simulink model "CDC2025_HybridAutomaton"  (R2023b)
settings: Solver=VariableStepAuto  StartTime=0.0  StopTime=sim_T  MaxStep=MaxStep  RelTol=RelTol
values from neighbouring files (symbols this model uses):
  A_sim = double(jacobian(dx, x))    [Settings_Simulation.m]
  B_sim = double(jacobian(dx, ui))    [Settings_Simulation.m]
  sim_T = 10    [MAIN_Simulation.m]
undefined symbols (not defined in the file or in its folder): control, leader, model, simulation
libraries: HyEQ_Library x1
settings Model: Creator=20155555  LastModifiedBy=20155555
settings OptimizationCC: BlockReduction=off  DefaultParameterBehavior=Inlined  BufferReuse=off

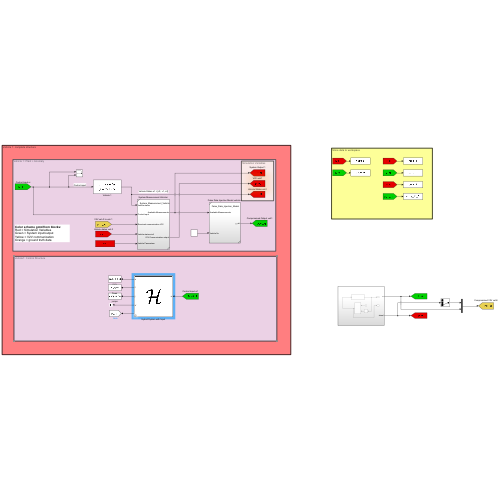
[thumbnail: Simulink's stored preview of the top-level diagram]
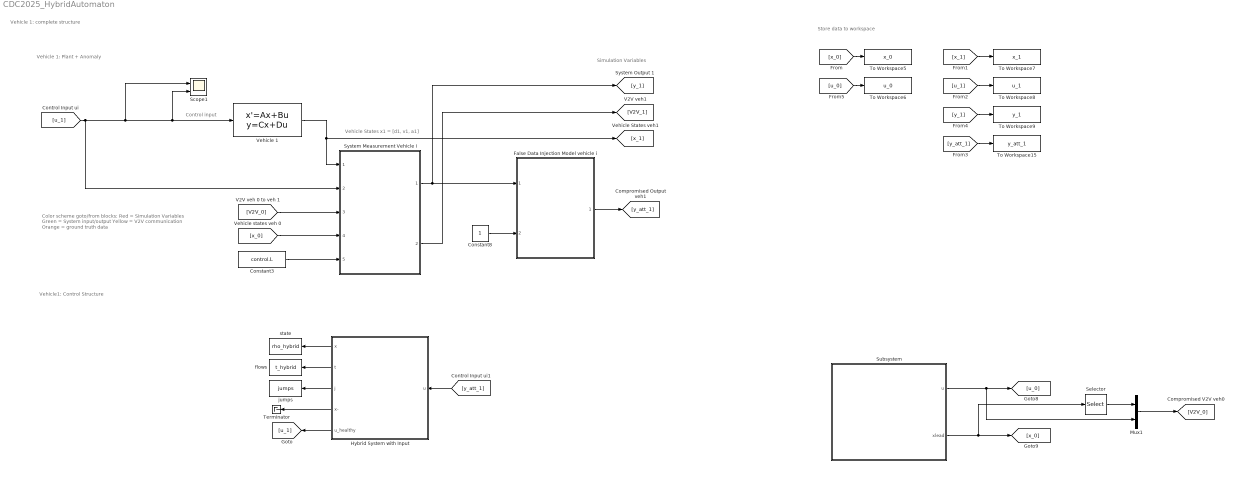
== system CDC2025_HybridAutomaton ==
  note: Vehicle 1: complete structure
  note: Vehicle1: Control Structure
  note: Vehicle States x1 = [d1, v1, a1]
  note: Store data to workspace
  note: Control input
  note: Vehicle 1: Plant + Anomaly
  note: Simulation Variables
  note: Color scheme goto/from blocks:
      | Red = Simulation Variables
      | Green = System input/output
      | Yellow = V2V communication
      | Orange = ground truth data
  Constant3 : Constant  Value=control.L
  Constant8 : Constant
  False Data Injection Model vehicle i : Subsystem  ReferencedSubsystem=False_Data_Injection_Model
  Hybrid System with Input : Subsystem  LoadFcn=set_param(gcb,'LinkStatus','none')  mask(Hybrid System with Inputs){x0=simulation.rho_init, input_dim=6, parameters=[control.h, model.tau, control.kp, control.kd, control.epsilon], T=sim_T, J=control.J, rule=Flow}
      mask prompts: x0 "Initial Condition (column vector)"; input_dim "Input Dimension (positive integer)"; T "Flow Horizon (nonnegative real)"; J "Jump Horizon (nonnegative integer)"; rule "Flow/Jump Priorty Rule"
      mask help:
      | To modify (f, g, C, D) for this block, "Look inside" the block mask by either clicking the down arrow in the lower-left corner or selecting "Mask" > "Look Under Mask" from the context menu.
      |
      | For instructions how to use this block, see the
      mask init:
      | state_dim = numel(x0);
      settings: CopyFcn=|
      | set_param(gcb,'LinkStatus','none'),
      | set_param(gcs, 'MaxStep', 'MaxStep', 'RelTol', 'RelTol','StopTime', 'T')
      mask Help:
      | To modify (f, g, C, D) for this block, "Look inside" the block mask by either clicking the down arrow in the lower-left corner or selecting "Mask" > "Look Under Mask" from the context menu.
      | 
      | The value given in the 'parameters' field is passed as the last input argument for f, g, C, and D. Any MATLAB object can be used, but we recommend using a struct. For example, in the initialization script, a parameters struct can be defined as followed.
      |   parameters = struct();
      |   parameters.A = eye(2);
      |   parameters.B = [1; 0];
      | 
      | The output "x-" is the state output delayed by one integration step. Use this output to break algebraic loops.
      mask TypeOptions x0: Integrator System/x0
      mask TypeOptions T: Integrator System/T
      mask TypeOptions J: Integrator System/J
      mask TypeOptions rule: Jump | Flow | Random
      mask DialogControl Control2 Prompt: Introduction to the HyEQ Simulink-based Library
      mask DialogControl Control2 Callback: hybrid.internal.openHelp('Help_SimulinkLibrary')
      mask DialogControl Container3 Prompt: System Configuration
      mask DialogControl Container2 Prompt: Solver Options
      mask Display:
      | image('Hcal.jpg')
      | port_label('output', 1, 'x')
      | port_label('output', 2, 't')
      | port_label('output', 3, 'j')
      | port_label('output', 4, 'x^-','texmode', 'on')
      | port_label('input', 1, 'u')
  Mux1 : Mux  Inputs=2
  Scope1 : Scope  NumInputPorts=2
  Selector : Selector  InputPortWidth=3  IndexOptions=Index vector (dialog)  Indices=[3]  OutputSizes=1
  Subsystem : Subsystem
  System Measurement Vehicle i : Subsystem  ReferencedSubsystem=System_Measurement_Vehicle
  Terminator : Terminator
  To Workspace15 : ToWorkspace  VariableName=y_att_1  SampleTime=-1
  To Workspace5 : ToWorkspace  VariableName=x_0  SampleTime=-1
  To Workspace6 : ToWorkspace  VariableName=u_0  SampleTime=-1
  To Workspace7 : ToWorkspace  VariableName=x_1  SampleTime=-1
  To Workspace8 : ToWorkspace  VariableName=u_1  SampleTime=-1
  To Workspace9 : ToWorkspace  VariableName=y_1  SampleTime=-1
  Vehicle 1 : StateSpace  A=A_sim  B=B_sim  C=eye(3)  D=zeros(3,1)  InitialCondition=simulation.veh1.x_init
  flows : ToWorkspace  VariableName=t_hybrid  SampleTime=-1
  jumps : ToWorkspace  VariableName=jumps  SampleTime=-1
  state : ToWorkspace  VariableName=rho_hybrid  SampleTime=-1
  wires:
  Hybrid System with Input/4(x-) -> Terminator/1
  Hybrid System with Input/1(x) -> state/1
  Hybrid System with Input/2(t) -> flows/1
  Hybrid System with Input/3(j) -> jumps/1
  Hybrid System with Input/5(u_healthy) -> [u_1]
  Constant8/1 -> False Data Injection Model vehicle i/2
  False Data Injection Model vehicle i/1 -> [y_att_1]
  [V2V_0] -> System Measurement Vehicle i/3
  [x_0] -> To Workspace5/1
  [y_att_1] -> To Workspace15/1
  Mux1/1 -> [V2V_0]
  [u_1] -> To Workspace8/1
  [x_1] -> To Workspace7/1
  [y_1] -> To Workspace9/1
  System Measurement Vehicle i/2 -> [V2V_1]
  [x_0] -> System Measurement Vehicle i/4
  [u_1] -> Vehicle 1/1, Scope1/2, Scope1/1, System Measurement Vehicle i/2
  Subsystem/2(xlead) -> Selector/1, [x_0]
  [u_0] -> To Workspace6/1
  Subsystem/1(u) -> Mux1/2, [u_0]
  Selector/1 -> Mux1/1
  Vehicle 1/1 -> System Measurement Vehicle i/1, [x_1]
  Constant3/1 -> System Measurement Vehicle i/5
  System Measurement Vehicle i/1 -> [y_1], False Data Injection Model vehicle i/1
  [y_att_1] -> Hybrid System with Input/1(u)

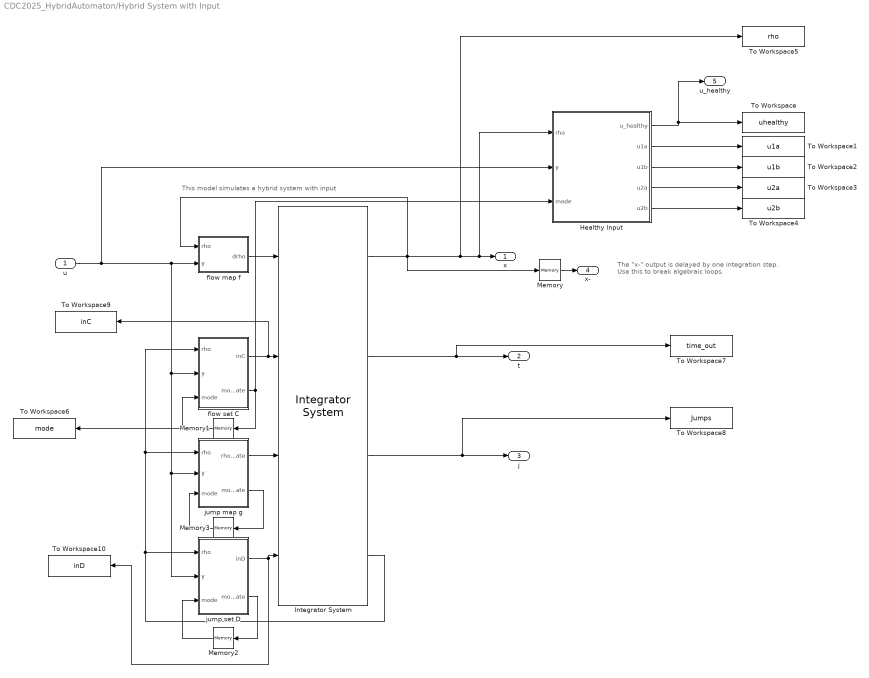
== system CDC2025_HybridAutomaton/Hybrid System with Input ==
  note: This model simulates a hybrid system with input
  note: The "x-" output is delayed by one integration step. Use this to break algebraic loops.
  u : Inport  PortDimensions=input_dim
  Healthy Input : MATLAB Function  TreatAsAtomicUnit=on
  Integrator System : HyEQ_Library/Other/Integrator System  Priority=2  T=T  J=J  x0=x0  rule=rule
      settings: SourceProductName=Hybrid Equations Toolbox
  Memory : Memory  InitialCondition=x0
  Memory1 : Memory  InheritSampleTime=on
  Memory2 : Memory  InheritSampleTime=on
  Memory3 : Memory  InheritSampleTime=on
  To Workspace : ToWorkspace  VariableName=uhealthy  SampleTime=-1
  To Workspace1 : ToWorkspace  VariableName=u1a  SampleTime=-1
  To Workspace10 : ToWorkspace  VariableName=inD  SampleTime=-1
  To Workspace2 : ToWorkspace  VariableName=u1b  SampleTime=-1
  To Workspace3 : ToWorkspace  VariableName=u2a  SampleTime=-1
  To Workspace4 : ToWorkspace  VariableName=u2b  SampleTime=-1
  To Workspace5 : ToWorkspace  VariableName=rho  SampleTime=-1
  To Workspace6 : ToWorkspace  VariableName=mode  SampleTime=-1
  To Workspace7 : ToWorkspace  VariableName=time_out  SampleTime=-1
  To Workspace8 : ToWorkspace  VariableName=Jumps  SampleTime=-1
  To Workspace9 : ToWorkspace  VariableName=inC  SampleTime=-1
  flow map f : MATLAB Function  TreatAsAtomicUnit=on
  flow set C : MATLAB Function  TreatAsAtomicUnit=on
  jump map g : MATLAB Function  TreatAsAtomicUnit=on
  jump set D : MATLAB Function  TreatAsAtomicUnit=on
  x : Outport  PortDimensions=state_dim
  t : Outport  Port=2  PortDimensions=1
  j : Outport  Port=3  PortDimensions=1
  x- : Outport  Port=4  PortDimensions=state_dim
  u_healthy : Outport  Port=5
  wires:
  Memory/1 -> x-/1
  jump map g/1(rho_update) -> Integrator System/3
  jump set D/1(inD) -> Integrator System/4, To Workspace10/1
  u/1 -> Healthy Input/2(y), jump set D/2(y), jump map g/2(y), flow set C/2(y), flow map f/2(y)
  Integrator System/3 -> To Workspace8/1, j/1
  Integrator System/2 -> To Workspace7/1, t/1
  flow set C/1(inC) -> To Workspace9/1, Integrator System/2
  Integrator System/1 -> flow map f/1(rho), To Workspace5/1, Healthy Input/1(rho), x/1, Memory/1
  Integrator System/4 -> flow set C/1(rho), jump map g/1(rho), jump set D/1(rho)
  flow map f/1(drho) -> Integrator System/1
  Memory1/1 -> flow set C/3(mode), To Workspace6/1
  Memory2/1 -> jump set D/3(mode)
  jump set D/2(mode_update) -> Memory2/1
  Memory3/1 -> jump map g/3(mode)
  jump map g/2(mode_update) -> Memory3/1
  Healthy Input/1(u_healthy) -> u_healthy/1, To Workspace/1
  Healthy Input/2(u1a) -> To Workspace1/1
  Healthy Input/5(u2b) -> To Workspace4/1
  Healthy Input/4(u2a) -> To Workspace3/1
  Healthy Input/3(u1b) -> To Workspace2/1
  flow set C/2(mode_update) -> Memory1/1, Healthy Input/3(mode)

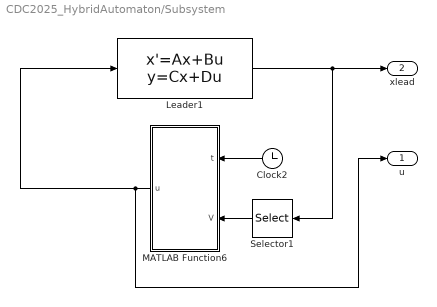
== system CDC2025_HybridAutomaton/Subsystem ==
  Clock2 : Clock
  Leader1 : StateSpace  A=A_sim  B=B_sim  C=eye(3)  D=zeros(3,1)  InitialCondition=simulation.veh0.x_init
  MATLAB Function6 : MATLAB Function  TreatAsAtomicUnit=on
  Selector1 : Selector  InputPortWidth=3  IndexOptions=Index vector (dialog)  Indices=2  OutputSizes=1
  u : Outport
  xlead : Outport  Port=2
  wires:
  Selector1/1 -> MATLAB Function6/2(V)
  MATLAB Function6/1(u) -> u/1, Leader1/1
  Leader1/1 -> xlead/1, Selector1/1
  Clock2/1 -> MATLAB Function6/1(t)

== matlab function CDC2025_HybridAutomaton/Subsystem/MATLAB Function6 ==
  data: t input; u output; V input; control parameter; leader parameter
function u = fcn(t, V, control, leader)


kp = control.kp;

Vdes = leader.Vdes0 ;
u = kp*(Vdes - V);

end

== matlab function CDC2025_HybridAutomaton/Hybrid System with Input/Healthy Input ==
  data: rho input size=state_dim; y input size=input_dim; mode input; u_healthy output size=1; parameters parameter; u1a output; u1b output; u2a output; u2b output
function [u_healthy, u1a, u1b, u2a, u2b]  = uHealthy(rho, y, mode, parameters)
% Define flow set indictor function here.

% allocate state
rho1a = rho(1);
rho1b = rho(2);
rho2a = rho(3);
rho2b = rho(4);

% Allocate output
y1 = y(1);
y2 = y(2);
y5a = y(3);
y5b = y(4);
y6a = y(5);
y6b = y(6);

% parameters
h = parameters(1);
tau = parameters(2);
kp = parameters(3);
kd = parameters(4);

% Compute control inputs before reset
u1a = compute_u1(y1, y2, y5a, rho1a, kd, h, tau);
u1b = compute_u1(y1, y2, y5b, rho1b, kd, h, tau);
u2a = compute_u2(y1, y2, rho2a, kd, h);
u2b = compute_u2(y1, y2, rho2b, kd, h);


if mode == 0
    u_healthy = u1a;
elseif mode ==  1
    u_healthy = u1b;
elseif mode == 2
    u_healthy = u1a;
elseif mode == 3
    u_healthy = u1a;
elseif mode == 4
    u_healthy = u1a;
else
    u_healthy = 69;
end

end



function u = compute_u1(y1, y2, y5, rho, kd, h, tau)
% Compute control input u1
u = rho + (kd/h) * y1 - kd * y2 + (tau/h) * y5;
end

function u = compute_u2(y1, y2, rho, kd, h)
% Compute control input u2
u = rho + (kd/h) * y1 - kd * y2;
end

== matlab function CDC2025_HybridAutomaton/Hybrid System with Input/flow map f ==
  data: rho input size=state_dim; y input size=input_dim; drho output size=state_dim; parameters parameter
function drho = f(rho, y, parameters)
% Define flow map here.

% parameters
h = parameters(1);
tau = parameters(2);
kp = parameters(3);
kd = parameters(4);

% States
rho1a = rho(1);
rho1b = rho(2);
rho2a = rho(3);
rho2b = rho(4);

% input
y1 = y(1);
y2 = y(2);
y5a = y(3);
y5b = y(4);
y6a = y(5);
y6b = y(6);

% Update states (flow dynamics)
drho1a = update_drho1(rho1a, y1, y2, y5a, h, kp, kd, tau);
drho1b = update_drho1(rho1b, y1, y2, y5b, h, kp, kd, tau);
drho2a = update_drho2(rho2a, y1, y2, y6a, h, kp, kd);
drho2b = update_drho2(rho2b, y1, y2, y6b, h, kp, kd);

drho = [drho1a; drho1b; drho2a; drho2b];

end


function drho = update_drho1(rho, y1, y2, y5, h, kp, kd, tau)
% Compute next state value
drho = (-1/h) * rho + (kp/h - kd/h^2) * y1 - (kp - kd/h) * y2 - (tau/h^2 - 1/h) * y5 - kp/h*3;
end

function drho = update_drho2(rho, y1, y2, y6, h, kp, kd)
% Compute next state value
drho = (-1/h) * rho + (kp/h - kd/h^2) * y1 - (kp - kd/h) * y2 + 1/h * y6 - kp/h*3;
end

== matlab function CDC2025_HybridAutomaton/Hybrid System with Input/flow set C ==
  data: rho input size=state_dim; y input size=input_dim; mode input; inC output size=1; parameters parameter; mode_update output
function [inC, mode_update] = C(rho, y, mode, parameters)
% Define flow set indictor function here.

% allocate state
rho1a = rho(1);
rho1b = rho(2);
rho2a = rho(3);
rho2b = rho(4);

% Allocate output
y1 = y(1);
y2 = y(2);
y5a = y(3);
y5b = y(4);
y6a = y(5);
y6b = y(6);

% parameters
h = parameters(1);
tau = parameters(2);
kp = parameters(3);
kd = parameters(4);
epsilon = parameters(5);

% Compute control inputs
u1a = compute_u1(y1, y2, y5a, rho1a, kd, h, tau);
u1b = compute_u1(y1, y2, y5b, rho1b, kd, h, tau);
u2a = compute_u2(y1, y2, rho2a, kd, h);
u2b = compute_u2(y1, y2, rho2b, kd, h);

% Determine transitions
[mode_update, inC, ~]  = get_next_mode(mode, u1a, u1b, u2a, u2b, y5a, y5b, y6a, y6b, rho1a, rho1b, rho2a, rho2b, h, tau, epsilon);



function [mode_update, inC, rho_update] = get_next_mode(mode, u1a, u1b, u2a, u2b, y5a, y5b, y6a, y6b, rho1a, rho1b, rho2a, rho2b, h, tau, epsilon)

% Compute next mode based on control inputs and state transitions
switch mode
    case 0
        if abs(u1a - u1b) > epsilon && abs(u1b - u2a) <= epsilon && abs(u2a - u2b) <= epsilon
            mode_update = 1;
            rho_update = [rho1a; rho1b; rho2a; rho2b];
            inC = false;
        elseif abs(u1b - u1a) > epsilon && abs(u1a - u2a) <= epsilon && abs(u2a - u2b) <= epsilon
            mode_update = 2;
            rho_update = [rho1a; rho1b; rho2a; rho2b];
            inC = false;
        elseif abs(u1a - u1b) <= epsilon && abs(u1b - u2b) <= epsilon && abs(u2b - u2a) > epsilon
            mode_update = 3;
            rho_update = [rho1a; rho1b; rho2a; rho2b];
            inC = false;
        elseif abs(u1a - u1b) <= epsilon && abs(u1b - u2a) <= epsilon && abs(u2a - u2b) > epsilon
            mode_update = 4;
            rho_update = [rho1a; rho1b; rho2a; rho2b];
            inC = false;
        else
            mode_update = mode;
            rho_update = [rho1a; rho1b; rho2a; rho2b];
            inC = true;
        end
    case 1 % Don't use u1a
        if abs(y5a - y5b) <= epsilon && abs(u1b - u2a) <= epsilon && abs(u2a - u2b) <= epsilon
            mode_update = 0;
            rho_update = [rho1b; rho1b; rho2a; rho2b];
            inC = false;
        elseif abs(u1b - u2a) > epsilon && abs(u2a - u2b) <= epsilon
            mode_update = 2;
            rho_update = [rho2a-tau/h*y5a; rho1b; rho2a; rho2b];
            inC = false;
        elseif abs(u1b - u2b) <= epsilon && abs(u2b - u2a) > epsilon
            mode_update = 3;
            rho_update = [rho1b; rho1b; rho2a; rho2b];
            % reset = 1;
            inC = false;
        elseif abs(u1b - u2a) <= epsilon && abs(u2a - u2b) > epsilon
            mode_update = 4;
            rho_update = [rho1b; rho1b; rho2a; rho2b];
            % reset = 1;
            inC = false;
        else
            mode_update = mode;
            rho_update = [rho1a; rho1b; rho2a; rho2b];
            inC = true;
        end
    case 2 % Don't use u1b
        if abs(y5a - y5b) <= epsilon && abs(u1a - u2a) <= epsilon && abs(u2a - u2b) <= epsilon
            mode_update = 0;
            rho_update = [rho1a; rho1a; rho2a; rho2b];
            inC = false;
        elseif abs(u1a - u2a) > epsilon && abs(u2a - u2b) <= epsilon
            mode_update = 1;
            rho_update = [rho1a; rho2a - tau/h*y5b; rho2a; rho2b];
            inC = false;
        elseif abs(u1a - u2a) > epsilon && abs(u1a - u2b) <= epsilon
            mode_update = 3;
            rho_update = [rho1a; rho1a; rho2a; rho2b];
            inC = false;
        elseif abs(u1a - u2a) <= epsilon && abs(u2a - u2b) > epsilon
            mode_update = 4;
            rho_update = [rho1a; rho1a; rho2a; rho2b];
            inC = false;
        else
            mode_update = mode;
            rho_update = [rho1a; rho1b; rho2a; rho2b];
            inC = true;
        end
    case 3 % Don't use u2a
        if abs(u1a - u1b) <= epsilon && abs(u1b - u2b) <= epsilon && abs(y6a - y6b) <= epsilon
            mode_update = 0;
            rho_update = [rho1a; rho1b; rho2b; rho2b];
            inC = false;
        elseif abs(u1a - u1b) > epsilon && abs(u1b - u2b) <= epsilon
            mode_update = 1;
            rho_update = [rho1a; rho1b; rho2b; rho2b];
            inC = false;
        elseif abs(u1b - u1a) > epsilon && abs(u1a - u2b) <= epsilon
            mode_update = 2;
            rho_update = [rho1a; rho1b; rho2b; rho2b];
            inC = false;
        elseif abs(u1a - u1b) <= epsilon && abs(u1b - u2b) > epsilon
            mode_update = 4;
            rho_update = [rho1a; rho1b; rho1a + tau/h*y5a; rho2b];
            inC = false;
        else
            mode_update = mode;
            rho_update = [rho1a; rho1b; rho2a; rho2b];
            inC = true;
        end
    case 4 % Don't use u2b
        if abs(u1a - u1b) <= epsilon && abs(u1b - u2a) <= epsilon && abs(y6a - y6b) <= epsilon
            mode_update = 0;
            rho_update = [rho1a; rho1b; rho2a; rho2a];
            inC = false;
        elseif abs(u1a - u1b) > epsilon && abs(u1b - u2a) <= epsilon
            mode_update = 1;
            rho_update = [rho1a; rho1b; rho2a; rho2a];
            inC = false;
        elseif abs(u1a - u1b) > epsilon && abs(u1a - u2a) <= epsilon
            mode_update = 2;
            rho_update = [rho1a; rho1b; rho2a; rho2a];
            inC = false;
        elseif abs(u1a - u1b) <= epsilon && abs(u1b - u2a) > epsilon
            mode_update = 3;
            rho_update = [rho1a; rho1b; rho2a; rho1a + tau/h*y5a];
            inC = false;
        else
            mode_update = mode;
            rho_update = [rho1a; rho1b; rho2a; rho2b];
            inC = true;
        end
    otherwise
        mode_update  = 69;
        rho_update = [0; 0; 0; 0];
        inC = true;
end
end

function u = compute_u1(y1, y2, y5, rho, kd, h, tau)
% Compute control input u1
u = rho + (kd/h) * y1 - kd * y2 + (tau/h) * y5;
end

function u = compute_u2(y1, y2, rho, kd, h)
% Compute control input u2
u = rho + (kd/h) * y1 - kd * y2;
end
end

== matlab function CDC2025_HybridAutomaton/Hybrid System with Input/jump map g ==
  data: rho input size=state_dim; y input size=input_dim; mode input; rho_update output size=state_dim; parameters parameter; mode_update output
function [rho_update, mode_update] = g(rho, y, mode, parameters)
% Jump map.

% allocate state
rho1a = rho(1);
rho1b = rho(2);
rho2a = rho(3);
rho2b = rho(4);

% Allocate output
y1 = y(1);
y2 = y(2);
y5a = y(3);
y5b = y(4);
y6a = y(5);
y6b = y(6);

% parameters
h = parameters(1);
tau = parameters(2);
kp = parameters(3);
kd = parameters(4);
epsilon = parameters(5);


% Compute control inputs
u1a = compute_u1(y1, y2, y5a, rho1a, kd, h, tau);
u1b = compute_u1(y1, y2, y5b, rho1b, kd, h, tau);
u2a = compute_u2(y1, y2, rho2a, kd, h);
u2b = compute_u2(y1, y2, rho2b, kd, h);

% Determine transitions
[mode_update, ~, rho_update]  = get_next_mode(mode, u1a, u1b, u2a, u2b, y5a, y5b, y6a, y6b, rho1a, rho1b, rho2a, rho2b, h, tau, epsilon);

end

function [mode_update, inD, rho_update] = get_next_mode(mode, u1a, u1b, u2a, u2b, y5a, y5b, y6a, y6b, rho1a, rho1b, rho2a, rho2b, h, tau, epsilon)

% Compute next mode based on control inputs and state transitions
switch mode
    case 0
        if abs(u1a - u1b) > epsilon && abs(u1b - u2a) <= epsilon && abs(u2a - u2b) <= epsilon
            mode_update = 1;
            rho_update = [rho1a; rho1b; rho2a; rho2b];
            inD = true;
        elseif abs(u1b - u1a) > epsilon && abs(u1a - u2a) <= epsilon && abs(u2a - u2b) <= epsilon
            mode_update = 2;
            rho_update = [rho1a; rho1b; rho2a; rho2b];
            inD = true;
        elseif abs(u1a - u1b) <= epsilon && abs(u1b - u2b) <= epsilon && abs(u2b - u2a) > epsilon
            mode_update = 3;
            rho_update = [rho1a; rho1b; rho2a; rho2b];
            inD = true;
        elseif abs(u1a - u1b) <= epsilon && abs(u1b - u2a) <= epsilon && abs(u2a - u2b) > epsilon
            mode_update = 4;
            rho_update = [rho1a; rho1b; rho2a; rho2b];
            inD = true;
        else
            mode_update = mode;
            rho_update = [rho1a; rho1b; rho2a; rho2b];
            inD = false;
        end
    case 1 % Don't use u1a
        if abs(y5a - y5b) <= epsilon && abs(u1b - u2a) <= epsilon && abs(u2a - u2b) <= epsilon
            mode_update = 0;
            rho_update = [rho1b; rho1b; rho2a; rho2b];
            inD = true;
        elseif abs(u1b - u2a) > epsilon && abs(u2a - u2b) <= epsilon
            mode_update = 2;
            rho_update = [rho2a-tau/h*y5a; rho1b; rho2a; rho2b];
            inD = true;
        elseif abs(u1b - u2b) <= epsilon && abs(u2b - u2a) > epsilon
            mode_update = 3;
            rho_update = [rho1b; rho1b; rho2a; rho2b];
            % reset = 1;
            inD = true;
        elseif abs(u1b - u2a) <= epsilon && abs(u2a - u2b) > epsilon
            mode_update = 4;
            rho_update = [rho1b; rho1b; rho2a; rho2b];
            % reset = 1;
            inD = true;
        else
            mode_update = mode;
            rho_update = [rho1a; rho1b; rho2a; rho2b];
            inD = false;
        end
    case 2 % Don't use u1b
        if abs(y5a - y5b) <= epsilon && abs(u1a - u2a) <= epsilon && abs(u2a - u2b) <= epsilon
            mode_update = 0;
            rho_update = [rho1a; rho1a; rho2a; rho2b];
            inD = true;
        elseif abs(u1a - u2a) > epsilon && abs(u2a - u2b) <= epsilon
            mode_update = 1;
            rho_update = [rho1a; rho2a - tau/h*y5b; rho2a; rho2b];
            inD = true;
        elseif abs(u1a - u2a) > epsilon && abs(u1a - u2b) <= epsilon
            mode_update = 3;
            rho_update = [rho1a; rho1a; rho2a; rho2b];
            inD = true;
        elseif abs(u1a - u2a) <= epsilon && abs(u2a - u2b) > epsilon
            mode_update = 4;
            rho_update = [rho1a; rho1a; rho2a; rho2b];
            inD = true;
        else
            mode_update = mode;
            rho_update = [rho1a; rho1b; rho2a; rho2b];
            inD = false;
        end
    case 3 % Don't use u2a
        if abs(u1a - u1b) <= epsilon && abs(u1b - u2b) <= epsilon && abs(y6a - y6b) <= epsilon
            mode_update = 0;
            rho_update = [rho1a; rho1b; rho2b; rho2b];
            inD = true;
        elseif abs(u1a - u1b) > epsilon && abs(u1b - u2b) <= epsilon
            mode_update = 1;
            rho_update = [rho1a; rho1b; rho2b; rho2b];
            inD = true;
        elseif abs(u1b - u1a) > epsilon && abs(u1a - u2b) <= epsilon
            mode_update = 2;
            rho_update = [rho1a; rho1b; rho2b; rho2b];
            inD = true;
        elseif abs(u1a - u1b) <= epsilon && abs(u1b - u2b) > epsilon
            mode_update = 4;
            rho_update = [rho1a; rho1b; rho1a + tau/h*y5a; rho2b];
            inD = true;
        else
            mode_update = mode;
            rho_update = [rho1a; rho1b; rho2a; rho2b];
            inD = true;
        end
    case 4 % Don't use u2b
        if abs(y5a - y5b) <= epsilon && abs(y6a - y6b) <= epsilon
            mode_update = 0;
            rho_update = [rho1a; rho1b; rho2a; rho2a];
            inD = true;
        elseif abs(u1a - u1b) > epsilon && abs(u1b - u2a) <= epsilon
            mode_update = 1;
            rho_update = [rho1a; rho1b; rho2a; rho2a];
            inD = true;
        elseif abs(u1a - u1b) > epsilon && abs(u1a - u2a) <= epsilon
            mode_update = 2;
            rho_update = [rho1a; rho1b; rho2a; rho2a];
            inD = true;
        elseif abs(u1a - u1b) <= epsilon && abs(u1b - u2a) > epsilon
            mode_update = 3;
            rho_update = [rho1a; rho1b; rho2a; rho1a + tau/h*y5a];
            inD = true;
        else
            mode_update = mode;
            rho_update = [rho1a; rho1b; rho2a; rho2b];
            inD = false;

        end
    otherwise
        mode_update  = 69;
        rho_update = [0; 0; 0; 0];
        inD = false;
end
end

function u = compute_u1(y1, y2, y5, rho, kd, h, tau)
% Compute control input u1
u = rho + (kd/h) * y1 - kd * y2 + (tau/h) * y5;
end

function u = compute_u2(y1, y2, rho, kd, h)
% Compute control input u2
u = rho + (kd/h) * y1 - kd * y2;
end

== matlab function CDC2025_HybridAutomaton/Hybrid System with Input/jump set D ==
  data: rho input size=state_dim; y input size=input_dim; mode input; inD output size=1; parameters parameter; mode_update output
function [inD, mode_update] = D(rho, y, mode, parameters)
% Define jump set indictor function here.

% allocate state
rho1a = rho(1);
rho1b = rho(2);
rho2a = rho(3);
rho2b = rho(4);

% Allocate output
y1 = y(1);
y2 = y(2);
y5a = y(3);
y5b = y(4);
y6a = y(5);
y6b = y(6);

% parameters
h = parameters(1);
tau = parameters(2);
kp = parameters(3);
kd = parameters(4);
epsilon = parameters(5);

% Compute control inputs
u1a = compute_u1(y1, y2, y5a, rho1a, kd, h, tau);
u1b = compute_u1(y1, y2, y5b, rho1b, kd, h, tau);
u2a = compute_u2(y1, y2, rho2a, kd, h);
u2b = compute_u2(y1, y2, rho2b, kd, h);

% Determine transitions
[mode_update, inD, ~]  = get_next_mode(mode, u1a, u1b, u2a, u2b, y5a, y5b, y6a, y6b, rho1a, rho1b, rho2a, rho2b, h, tau, epsilon);



function [mode_update, inD, rho_update] = get_next_mode(mode, u1a, u1b, u2a, u2b, y5a, y5b, y6a, y6b, rho1a, rho1b, rho2a, rho2b, h, tau, epsilon)

% Compute next mode based on control inputs and state transitions
switch mode
    case 0
        if abs(u1a - u1b) > epsilon && abs(u1b - u2a) <= epsilon && abs(u2a - u2b) <= epsilon
            mode_update = 1;
            rho_update = [rho1a; rho1b; rho2a; rho2b];
            inD = true;
        elseif abs(u1b - u1a) > epsilon && abs(u1a - u2a) <= epsilon && abs(u2a - u2b) <= epsilon
            mode_update = 2;
            rho_update = [rho1a; rho1b; rho2a; rho2b];
            inD = true;
        elseif abs(u1a - u1b) <= epsilon && abs(u1b - u2b) <= epsilon && abs(u2b - u2a) > epsilon
            mode_update = 3;
            rho_update = [rho1a; rho1b; rho2a; rho2b];
            inD = true;
        elseif abs(u1a - u1b) <= epsilon && abs(u1b - u2a) <= epsilon && abs(u2a - u2b) > epsilon
            mode_update = 4;
            rho_update = [rho1a; rho1b; rho2a; rho2b];
            inD = true;
        else
            mode_update = mode;
            rho_update = [rho1a; rho1b; rho2a; rho2b];
            inD = false;
        end
    case 1 % Don't use u1a
        if abs(y5a - y5b) <= epsilon && abs(u1b - u2a) <= epsilon && abs(u2a - u2b) <= epsilon
            mode_update = 0;
            rho_update = [rho1b; rho1b; rho2a; rho2b];
            inD = true;
        elseif abs(u1b - u2a) > epsilon && abs(u2a - u2b) <= epsilon
            mode_update = 2;
            rho_update = [rho2a-tau/h*y5a; rho1b; rho2a; rho2b];
            inD = true;
        elseif abs(u1b - u2b) <= epsilon && abs(u2b - u2a) > epsilon
            mode_update = 3;
            rho_update = [rho1b; rho1b; rho2a; rho2b];
            % reset = 1;
            inD = true;
        elseif abs(u1b - u2a) <= epsilon && abs(u2a - u2b) > epsilon
            mode_update = 4;
            rho_update = [rho1b; rho1b; rho2a; rho2b];
            % reset = 1;
            inD = true;
        else
            mode_update = mode;
            rho_update = [rho1a; rho1b; rho2a; rho2b];
            inD = false;
        end
    case 2 % Don't use u1b
        if abs(y5a - y5b) <= epsilon && abs(u1a - u2a) <= epsilon && abs(u2a - u2b) <= epsilon
            mode_update = 0;
            rho_update = [rho1a; rho1a; rho2a; rho2b];
            inD = true;
        elseif abs(u1a - u2a) > epsilon && abs(u2a - u2b) <= epsilon
            mode_update = 1;
            rho_update = [rho1a; rho2a - tau/h*y5b; rho2a; rho2b];
            inD = true;
        elseif abs(u1a - u2a) > epsilon && abs(u1a - u2b) <= epsilon
            mode_update = 3;
            rho_update = [rho1a; rho1a; rho2a; rho2b];
            inD = true;
        elseif abs(u1a - u2a) <= epsilon && abs(u2a - u2b) > epsilon
            mode_update = 4;
            rho_update = [rho1a; rho1a; rho2a; rho2b];
            inD = true;
        else
            mode_update = mode;
            rho_update = [rho1a; rho1b; rho2a; rho2b];
            inD = false;
        end
    case 3 % Don't use u2a
        if abs(u1a - u1b) <= epsilon && abs(u1b - u2b) <= epsilon && abs(y6a - y6b) <= epsilon
            mode_update = 0;
            rho_update = [rho1a; rho1b; rho2b; rho2b];
            inD = true;
        elseif abs(u1a - u1b) > epsilon && abs(u1b - u2b) <= epsilon
            mode_update = 1;
            rho_update = [rho1a; rho1b; rho2b; rho2b];
            inD = true;
        elseif abs(u1b - u1a) > epsilon && abs(u1a - u2b) <= epsilon
            mode_update = 2;
            rho_update = [rho1a; rho1b; rho2b; rho2b];
            inD = true;
        elseif abs(u1a - u1b) <= epsilon && abs(u1b - u2b) > epsilon
            mode_update = 4;
            rho_update = [rho1a; rho1b; rho1a + tau/h*y5a; rho2b];
            inD = true;
        else
            mode_update = mode;
            rho_update = [rho1a; rho1b; rho2a; rho2b];
            inD = false;
        end
    case 4 % Don't use u2b
        if abs(u1a - u1b) <= epsilon && abs(u1b - u2a) <= epsilon && abs(y6a - y6b) <= epsilon
            mode_update = 0;
            rho_update = [rho1a; rho1b; rho2a; rho2a];
            inD = true;
        elseif abs(u1a - u1b) > epsilon && abs(u1b - u2a) <= epsilon
            mode_update = 1;
            rho_update = [rho1a; rho1b; rho2a; rho2a];
            inD = true;
        elseif abs(u1a - u1b) > epsilon && abs(u1a - u2a) <= epsilon
            mode_update = 2;
            rho_update = [rho1a; rho1b; rho2a; rho2a];
            inD = true;
        elseif abs(u1a - u1b) <= epsilon && abs(u1b - u2a) > epsilon
            mode_update = 3;
            rho_update = [rho1a; rho1b; rho2a; rho1a + tau/h*y5a];
            inD = true;
        else
            mode_update = mode;
            rho_update = [rho1a; rho1b; rho2a; rho2b];
            inD = false;

        end
    otherwise
        mode_update  = 69;
        rho_update = [0; 0; 0; 0];
        inD = false;
end
end

function u = compute_u1(y1, y2, y5, rho, kd, h, tau)
% Compute control input u1
u = rho + (kd/h) * y1 - kd * y2 + (tau/h) * y5;
end

function u = compute_u2(y1, y2, rho, kd, h)
% Compute control input u2
u = rho + (kd/h) * y1 - kd * y2;
end
end
